simulink model "Batery_Model"  (R2016b)
settings: Solver=VariableStepAuto  StartTime=0.0  StopTime=9.759939900040627e+04  RelTol=10  AbsTol=10
values from neighbouring files (symbols this model uses):
  R0 = Average_R0(meas.Current,meas.Voltage)    [Copy_of_generate_dynamic_parameters_relaxation.m]    (also in Optimization.m = vOpt(5).Value; Semi-Automatic Li Ion battery  RC model parameters estimator.m = vOpt(5).Value; generate_dynamic_parameters_relaxation.m = Average_R0(meas.Current, meas.Voltage))
libraries: fl_lib x5, nesl_utility x5
settings Model: Creator=Fededc88  LastModifiedBy=Fededc88

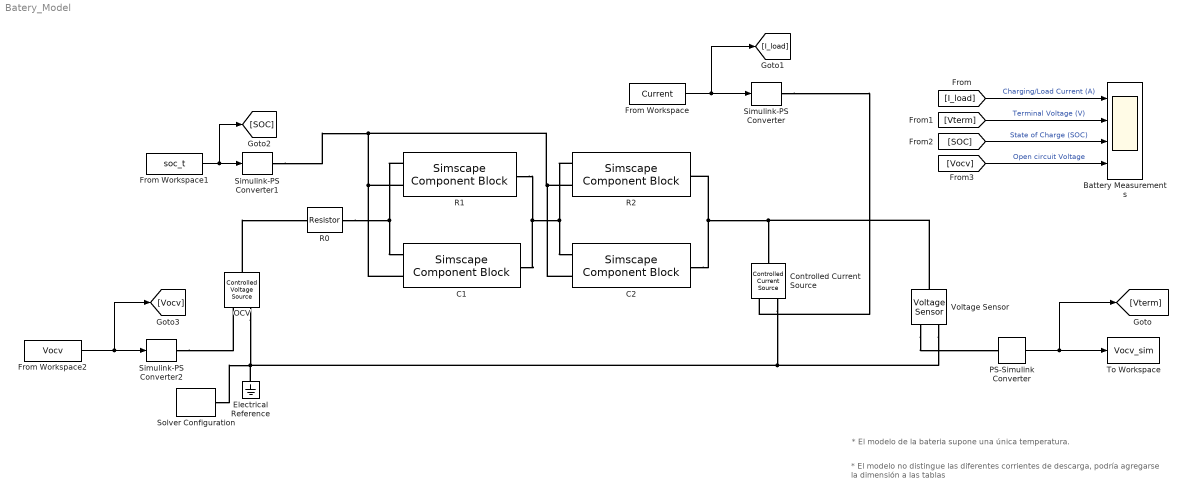
== system Batery_Model ==
  note: * El modelo no distingue las diferentes corrientes de descarga,
      | podría agregarse la dimensión a las tablas
  note: * El modelo de la bateria supone una única temperatura.
  Battery Measurements : Scope  NumInputPorts=4
  C1 : SimscapeComponentBlock  SourceFile=C_table_1Temp  ComponentPath=C_table_1Temp  ComponentVariants=C_table_1Temp  ComponentVariantNames=C_table_1Temp  ClassName=C_table_1Temp  SchemaVersion=1  C_Table=C1_table F  SOC_Table=SOC_table  v0=0 V
      settings: CopyFcn=simscape.engine.sli.internal.componentblockcallback(gcbh,'COPY')  PreCopyFcn=simscape.engine.sli.internal.componentblockcallback(gcbh,'PRECOPY')  PreDeleteFcn=simscape.engine.sli.internal.componentblockcallback(gcbh,'PREDELETE')
      mask Type: C_table_1Temp
      mask Display:
      | disp('Simscape\n\n\n')
      | disp('\n\n\nC_table_1Temp');
      | color('red');
      | port_label('LConn', 2,'SOC');
      | port_label('RConn', 1,'-');
      | port_label('LConn', 1,'+');
  C2 : SimscapeComponentBlock  SourceFile=C_table_1Temp  ComponentPath=C_table_1Temp  ComponentVariants=C_table_1Temp  ComponentVariantNames=C_table_1Temp  ClassName=C_table_1Temp  SchemaVersion=1  C_Table=C2_table F  SOC_Table=SOC_table  v0=0 V
      settings: CopyFcn=simscape.engine.sli.internal.componentblockcallback(gcbh,'COPY')  PreCopyFcn=simscape.engine.sli.internal.componentblockcallback(gcbh,'PRECOPY')  PreDeleteFcn=simscape.engine.sli.internal.componentblockcallback(gcbh,'PREDELETE')
      mask Type: C_table_1Temp
      mask Display:
      | disp('Simscape\n\n\n')
      | disp('\n\n\nC_table_1Temp');
      | color('red');
      | port_label('LConn', 2,'SOC');
      | port_label('RConn', 1,'-');
      | port_label('LConn', 1,'+');
  Controlled Current Source : fl_lib/Electrical/Electrical Sources/Controlled Current Source
  Electrical Reference : fl_lib/Electrical/Electrical Elements/Electrical Reference
  From Workspace : FromWorkspace  VariableName=Current  OutDataTypeStr=double  SampleTime=0
  From Workspace1 : FromWorkspace  VariableName=soc_t  SampleTime=0
  From Workspace2 : FromWorkspace  VariableName=Vocv  SampleTime=0
  OCV : fl_lib/Electrical/Electrical Sources/Controlled Voltage Source
  PS-Simulink Converter : nesl_utility/PS-Simulink Converter  PhysicalDomain=network_engine_domain  SubClassName=ps_output  LeftPortType=input  RightPortType=output  PseudoPeriodic=off  Frequencies=[]  Unit=V  AffineConversion=off
  R0 : fl_lib/Electrical/Electrical Elements/Resistor  R=R0 Ohm  i_specify=off  i_priority=None  i=0 A  v_specify=off  v_priority=None  v=0 V
  R1 : SimscapeComponentBlock  SourceFile=R_table_1Temp  ComponentPath=R_table_1Temp  ComponentVariants=R_table_1Temp  ComponentVariantNames=R_table_1Temp  ClassName=R_table_1Temp  SchemaVersion=1  R_Table=R1_table Ohm  SOC_Table=SOC_table
      settings: CopyFcn=simscape.engine.sli.internal.componentblockcallback(gcbh,'COPY')  PreCopyFcn=simscape.engine.sli.internal.componentblockcallback(gcbh,'PRECOPY')  PreDeleteFcn=simscape.engine.sli.internal.componentblockcallback(gcbh,'PREDELETE')
      mask Type: R_table_1Temp
      mask Display:
      | disp('Simscape\n\n\n')
      | disp('\n\n\nR_table_1Temp');
      | color('red');
      | port_label('LConn', 2,'SOC');
      | port_label('RConn', 1,'-');
      | port_label('LConn', 1,'+');
  R2 : SimscapeComponentBlock  SourceFile=R_table_1Temp  ComponentPath=R_table_1Temp  ComponentVariants=R_table_1Temp  ComponentVariantNames=R_table_1Temp  ClassName=R_table_1Temp  SchemaVersion=1  R_Table=R2_table Ohm  SOC_Table=SOC_table
      settings: CopyFcn=simscape.engine.sli.internal.componentblockcallback(gcbh,'COPY')  PreCopyFcn=simscape.engine.sli.internal.componentblockcallback(gcbh,'PRECOPY')  PreDeleteFcn=simscape.engine.sli.internal.componentblockcallback(gcbh,'PREDELETE')
      mask Type: R_table_1Temp
      mask Display:
      | disp('Simscape\n\n\n')
      | disp('\n\n\nR_table_1Temp');
      | color('red');
      | port_label('LConn', 2,'SOC');
      | port_label('RConn', 1,'-');
      | port_label('LConn', 1,'+');
  Simulink-PS Converter : nesl_utility/Simulink-PS Converter  PhysicalDomain=network_engine_domain  SubClassName=ps_input  LeftPortType=input  RightPortType=output  PseudoPeriodic=off  Frequencies=[]  NoiseDistribution=none  NoiseParameters=[]  Unit=A  AffineConversion=off  InputFiltering=off  SimscapeFilterOrder=1  InputFilterTimeConstant=.001  UdotUserProvided=1
  Simulink-PS Converter1 : nesl_utility/Simulink-PS Converter  PhysicalDomain=network_engine_domain  SubClassName=ps_input  LeftPortType=input  RightPortType=output  PseudoPeriodic=off  Frequencies=[]  NoiseDistribution=none  NoiseParameters=[]  Unit=1  AffineConversion=on  InputFiltering=off  SimscapeFilterOrder=1  InputFilterTimeConstant=.001  UdotUserProvided=1
  Simulink-PS Converter2 : nesl_utility/Simulink-PS Converter  PhysicalDomain=network_engine_domain  SubClassName=ps_input  LeftPortType=input  RightPortType=output  PseudoPeriodic=off  Frequencies=[]  NoiseDistribution=none  NoiseParameters=[]  Unit=V  AffineConversion=off  InputFiltering=off  SimscapeFilterOrder=1  InputFilterTimeConstant=.001  UdotUserProvided=1
  Solver Configuration : nesl_utility/Solver Configuration  PhysicalDomain=network_engine_domain  SubClassName=solver  LeftPortType=input  RightPortType=generic  Accelerate=off  Tones=[]  Harmonics=[]  SimulateNoise=off  Profile=off  UseLocalSampling=off  EnableSwitchedLinearOptims=on  FrequencyDomain=off  UseCCode=off  RelTol=0.001  AbsTol=1e-06  MinStep=1e-09  ToWorkspace=off  RevertToSquareIcSolve=off  NumHomotopyIterations=100  PhasorMode=off  PhasorModeNumHarmonics=1  OverrideAbsTol=off  DoDC=off  ResidualTolerance=1  UseLocalSolver=on  LocalSolverChoice=NE_BACKWARD_EULER_ADVANCER  LocalSolverSampleTime=0.1  DoFixedCost=on  MaxNonlinIter=3  MaxModeIter=2  LinearAlgebra=Full  DelaysMemoryBudget=1024  AutomaticFiltering=off  FilteringTimeConstant=0.001
  To Workspace : ToWorkspace  VariableName=Vocv_sim  SaveFormat=Timeseries  SampleTime=-1
  Voltage Sensor : fl_lib/Electrical/Electrical Sensors/Voltage Sensor
  wires:
  PS-Simulink Converter/1 -> [Vterm], To Workspace/1
  From Workspace1/1 -> [SOC], Simulink-PS Converter1/1
  [SOC] -> Battery Measurements/3  "State of Charge (SOC)"
  [I_load] -> Battery Measurements/1  "Charging/Load Current (A)"
  [Vterm] -> Battery Measurements/2  "Terminal Voltage (V)"
  From Workspace2/1 -> [Vocv], Simulink-PS Converter2/1
  [Vocv] -> Battery Measurements/4  "Open circuit Voltage"
  From Workspace/1 -> [I_load], Simulink-PS Converter/1
  connections:
  R2/LConn1 -- R1/RConn1 -- C1/RConn1 -- C2/LConn1
  R1/LConn1 -- R0/RConn1 -- C1/LConn1
  C2/RConn1 -- Voltage Sensor/LConn1 -- Controlled Current Source/LConn1 -- R2/RConn1
  Electrical Reference/LConn1 -- Voltage Sensor/RConn2 -- Controlled Current Source/RConn2 -- OCV/RConn2 -- Solver Configuration/RConn1
  Voltage Sensor/RConn1 -- PS-Simulink Converter/LConn1
  Simulink-PS Converter1/RConn1 -- C2/LConn2 -- R2/LConn2 -- R1/LConn2 -- C1/LConn2
  OCV/LConn1 -- R0/LConn1
  Simulink-PS Converter2/RConn1 -- OCV/RConn1
  Simulink-PS Converter/RConn1 -- Controlled Current Source/RConn1
